simulink model "Lab3_PID"  (R2022a)
settings: Solver=VariableStepAuto  StartTime=0.0  StopTime=10.0  RelTol=1e-3
settings Model: Creator=bebawy  LastModifiedBy=bebawy

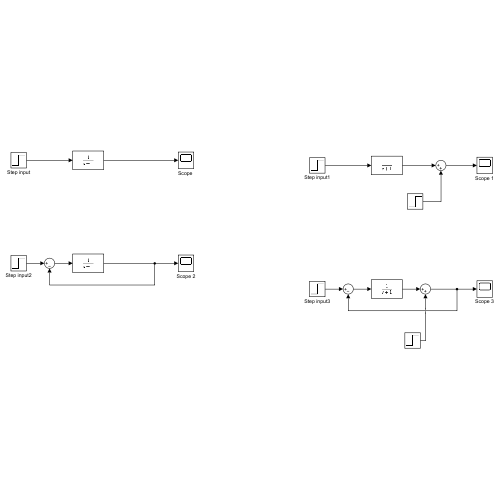
[thumbnail: Simulink's stored preview of the top-level diagram]
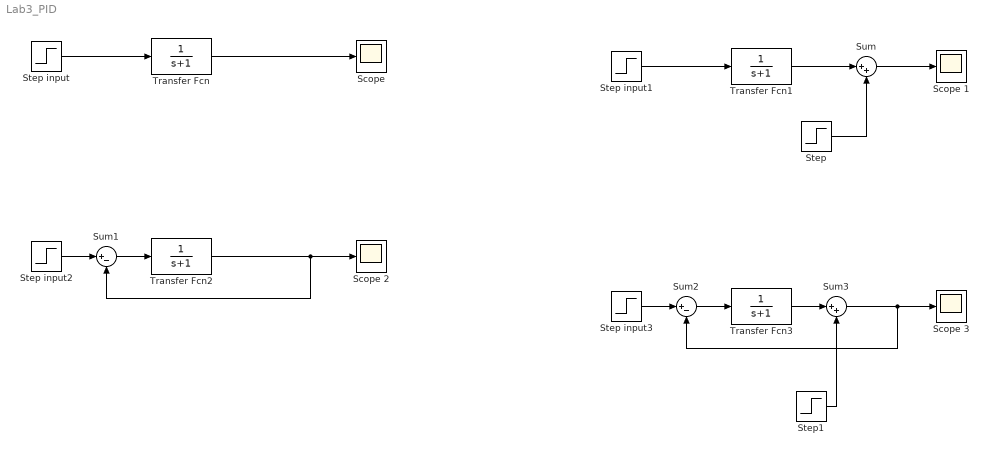
== system Lab3_PID ==
  Scope {,1..3} (4 alike) : Scope
  Step : Step  Time=3  SampleTime=0
  Step input{,1..3} (4 alike) : Step  SampleTime=0
  Step1 : Step  Time=3  SampleTime=0
  Sum : Sum  Inputs=|++
  Sum1 : Sum  Inputs=|+-
  Sum2 : Sum  Inputs=|+-
  Sum3 : Sum  Inputs=|++
  Transfer Fcn{,1..3} (4 alike) : TransferFcn  Denominator=[1 1]
  wires:
  Transfer Fcn/1 -> "Scope "/1
  Step input/1 -> Transfer Fcn/1
  Step input1/1 -> Transfer Fcn1/1
  Transfer Fcn1/1 -> Sum/1
  Sum/1 -> Scope 1/1
  Step/1 -> Sum/2
  Transfer Fcn2/1 -> Sum1/2, Scope 2/1
  Sum1/1 -> Transfer Fcn2/1
  Step input2/1 -> Sum1/1
  Step input3/1 -> Sum2/1
  Transfer Fcn3/1 -> Sum3/1
  Sum2/1 -> Transfer Fcn3/1
  Sum3/1 -> Sum2/2, Scope 3/1
  Step1/1 -> Sum3/2
